simulink model "Kalman_filter_Model"  (R2021b)
settings: Solver=VariableStepAuto  StartTime=0.0  StopTime=10  RelTol=1e-3
values from neighbouring files (symbols this model uses):
  A = [0 -6;1 -1]    [Kalman_filter_parameter.m]
  b = [1;0]    [Kalman_filter_parameter.m]
  C = [1 0]    [Kalman_filter_parameter.m]
  G = eye(2)    [Kalman_filter_parameter.m]
  L = K'    [Kalman_filter_parameter.m]
  V = 1    [Kalman_filter_parameter.m]
  W = [5 3;3 5]    [Kalman_filter_parameter.m]
libraries: simulink x3
settings Model: Creator=16970  LastModifiedBy=16970

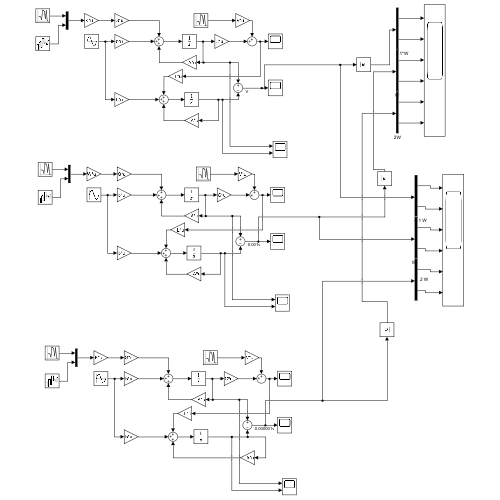
[thumbnail: Simulink's stored preview of the top-level diagram]
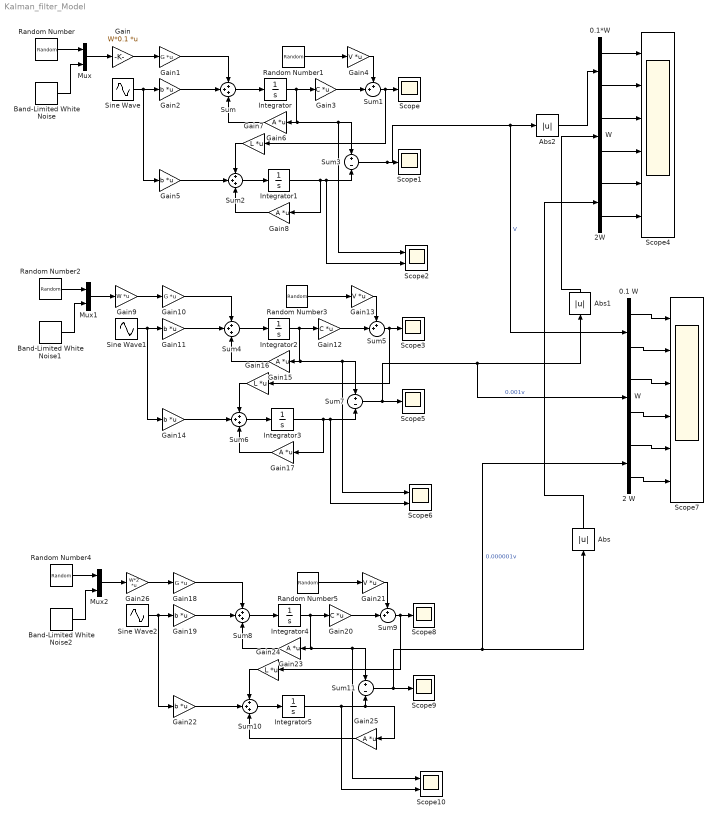
== system Kalman_filter_Model ==
  "\t0.1 W" : Demux  Outputs=2
  "\t0.1*W" : Demux  Outputs=2
  2 W : Demux  Outputs=2
  2W : Demux  Outputs=2
  Abs : Abs
  Abs1 : Abs
  Abs2 : Abs
  Band-Limited White Noise : simulink/Sources/Band-Limited White Noise  Cov=[0.1]  Ts=0.1  seed=[23341]
  Band-Limited White Noise1 : simulink/Sources/Band-Limited White Noise  Cov=[0.1]  Ts=0.1  seed=[23341]
  Band-Limited White Noise2 : simulink/Sources/Band-Limited White Noise  Cov=[0.1]  Ts=0.1  seed=[23341]
  Gain : Gain  Gain=W*0.1  Multiplication=Matrix(K*u)
  Gain1 : Gain  Gain=G  Multiplication=Matrix(K*u)
  Gain10 : Gain  Gain=G  Multiplication=Matrix(K*u)
  Gain{2,5,11,14,19,22} (6 alike) : Gain  Gain=b  Multiplication=Matrix(K*u)
  Gain12 : Gain  Gain=C  Multiplication=Matrix(K*u)
  Gain13 : Gain  Gain=V  Multiplication=Matrix(K*u)
  Gain{6,8,15,17,23,25} (6 alike) : Gain  Gain=A  Multiplication=Matrix(K*u)
  Gain16 : Gain  Gain=L  Multiplication=Matrix(K*u)
  Gain18 : Gain  Gain=G  Multiplication=Matrix(K*u)
  Gain20 : Gain  Gain=C  Multiplication=Matrix(K*u)
  Gain21 : Gain  Gain=V  Multiplication=Matrix(K*u)
  Gain24 : Gain  Gain=L  Multiplication=Matrix(K*u)
  Gain26 : Gain  Gain=W*2  Multiplication=Matrix(K*u)
  Gain3 : Gain  Gain=C  Multiplication=Matrix(K*u)
  Gain4 : Gain  Gain=V  Multiplication=Matrix(K*u)
  Gain7 : Gain  Gain=L  Multiplication=Matrix(K*u)
  Gain9 : Gain  Gain=W  Multiplication=Matrix(K*u)
  Integrator : Integrator  InitialCondition=[1;0]
  Integrator1 : Integrator  InitialCondition=[0;0]
  Integrator2 : Integrator  InitialCondition=[1;0]
  Integrator3 : Integrator  InitialCondition=[0;0]
  Integrator4 : Integrator  InitialCondition=[1;0]
  Integrator5 : Integrator  InitialCondition=[0;0]
  Mux : Mux  Inputs=2
  Mux1 : Mux  Inputs=2
  Mux2 : Mux  Inputs=2
  Random Number{,1..5} (6 alike) : RandomNumber  SampleTime=0.1
  Scope{,1,3,5,8..9} (6 alike) : Scope
  Scope10 : Scope  NumInputPorts=2
  Scope2 : Scope  NumInputPorts=2
  Scope4 : Scope  NumInputPorts=6
  Scope6 : Scope  NumInputPorts=2
  Scope7 : Scope  NumInputPorts=6
  Sine Wave : Sin  SampleTime=0
  Sine Wave1 : Sin  SampleTime=0
  Sine Wave2 : Sin  SampleTime=0
  Sum{,2,4,6,8,10} (6 alike) : Sum  Inputs=+++
  Sum1 : Sum  Inputs=++|
  Sum11 : Sum  Inputs=+|-
  Sum3 : Sum  Inputs=+|-
  Sum5 : Sum  Inputs=++|
  Sum7 : Sum  Inputs=+|-
  Sum9 : Sum  Inputs=++|
  W : Demux  Outputs=2
  "W   " : Demux  Outputs=2
  wires:
  Random Number/1 -> Mux/1
  Band-Limited White Noise/1 -> Mux/2
  Mux/1 -> Gain/1
  Gain/1 -> Gain1/1
  Gain1/1 -> Sum/1
  Sum/1 -> Integrator/1
  Integrator/1 -> Scope2/1, Sum3/1, Gain6/1, Gain3/1
  Gain3/1 -> Sum1/2
  Random Number1/1 -> Gain4/1
  Gain4/1 -> Sum1/1
  Sum1/1 -> Scope/1, Gain7/1
  Gain5/1 -> Sum2/2
  Sine Wave/1 -> Gain5/1, Gain2/1
  Sum2/1 -> Integrator1/1
  Integrator1/1 -> Gain8/1, Scope2/2, Sum3/2
  Gain6/1 -> Sum/3
  Gain7/1 -> Sum2/1
  Gain8/1 -> Sum2/3
  Sum3/1 -> "\t0.1 W"/1, Abs2/1, Scope1/1  "V"
  Gain2/1 -> Sum/2
  Gain11/1 -> Sum4/2
  Gain17/1 -> Sum6/3
  Band-Limited White Noise1/1 -> Mux1/2
  Gain14/1 -> Sum6/2
  Integrator2/1 -> Scope6/1, Sum7/1, Gain15/1, Gain12/1
  Gain16/1 -> Sum6/1
  Sum4/1 -> Integrator2/1
  Sum5/1 -> Scope3/1, Gain16/1
  Sum6/1 -> Integrator3/1
  Random Number3/1 -> Gain13/1
  Integrator3/1 -> Gain17/1, Scope6/2, Sum7/2
  Gain10/1 -> Sum4/1
  Sine Wave1/1 -> Gain14/1, Gain11/1
  Gain15/1 -> Sum4/3
  Mux1/1 -> Gain9/1
  Gain9/1 -> Gain10/1
  Random Number2/1 -> Mux1/1
  Gain13/1 -> Sum5/1
  Gain12/1 -> Sum5/2
  Sum7/1 -> "W   "/1, Abs1/1, Scope5/1  "0.001v"
  Sum10/1 -> Integrator5/1
  Sum9/1 -> Scope8/1, Gain24/1
  Gain24/1 -> Sum10/1
  Gain22/1 -> Sum10/2
  Integrator4/1 -> Scope10/1, Sum11/1, Gain23/1, Gain20/1
  Sum8/1 -> Integrator4/1
  Band-Limited White Noise2/1 -> Mux2/2
  Mux2/1 -> Gain26/1
  Gain23/1 -> Sum8/3
  Random Number5/1 -> Gain21/1
  Gain25/1 -> Sum10/3
  Sine Wave2/1 -> Gain22/1, Gain19/1
  Gain26/1 -> Gain18/1
  Random Number4/1 -> Mux2/1
  Gain20/1 -> Sum9/2
  Sum11/1 -> 2 W/1, Abs/1, Scope9/1  "0.000001v"
  Gain18/1 -> Sum8/1
  Gain21/1 -> Sum9/1
  Gain19/1 -> Sum8/2
  Integrator5/1 -> Gain25/1, Sum11/2, Scope10/2
  "\t0.1*W"/1 -> Scope4/1
  "\t0.1*W"/2 -> Scope4/2
  W/1 -> Scope4/3
  W/2 -> Scope4/4
  2W/1 -> Scope4/5
  2W/2 -> Scope4/6
  Abs/1 -> 2W/1
  Abs1/1 -> W/1
  Abs2/1 -> "\t0.1*W"/1
  2 W/1 -> Scope7/5
  "\t0.1 W"/2 -> Scope7/2
  "\t0.1 W"/1 -> Scope7/1
  "W   "/2 -> Scope7/4
  2 W/2 -> Scope7/6
  "W   "/1 -> Scope7/3
